simulink model "Simulink_1DOF_syst"  (R2016b)
settings: Solver=VariableStepAuto  StartTime=0.0  StopTime=10.0  RelTol=1e-3
undefined symbols (not defined in the file): c, k, m
settings Model: Creator=3700091  LastModifiedBy=3700091

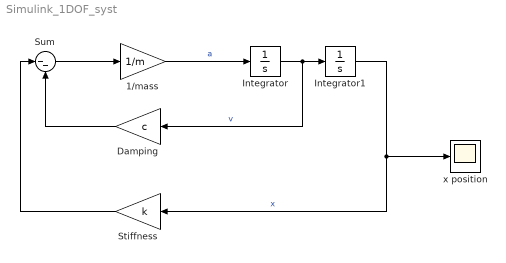
== system Simulink_1DOF_syst ==
  1/mass : Gain  Gain=1/m
  Damping : Gain  Gain=c
  Integrator : Integrator
  Integrator1 : Integrator
  Stiffness : Gain  Gain=k
  Sum : Sum  Inputs=|--
  x position : Scope
  wires:
  1/mass/1 -> Integrator/1  "a"
  Integrator/1 -> Damping/1, Integrator1/1  "v"
  Integrator1/1 -> x position/1, Stiffness/1  "x"
  Sum/1 -> 1/mass/1
  Damping/1 -> Sum/2
  Stiffness/1 -> Sum/1
